simulink subsystem "Subsystem_TugAzimuth"  (R2023a)
settings: Solver=VariableStepAuto  StartTime=0.0  StopTime=10.0  RelTol=1e-3
model mask{PosAz=0}
  mask prompts: PosAz "Coordinates of azimuth: [x;y]"
settings Model: Creator=henni  LastModifiedBy=rkr021
settings DebuggingCC: UnconnectedInputMsg=warning  UnconnectedOutputMsg=warning  UnconnectedLineMsg=warning
settings ModelReferenceCC: EnableRefExpFcnMdlSchedulingChecks=on
settings RTWCC: DLArmComputeVersion=19.05

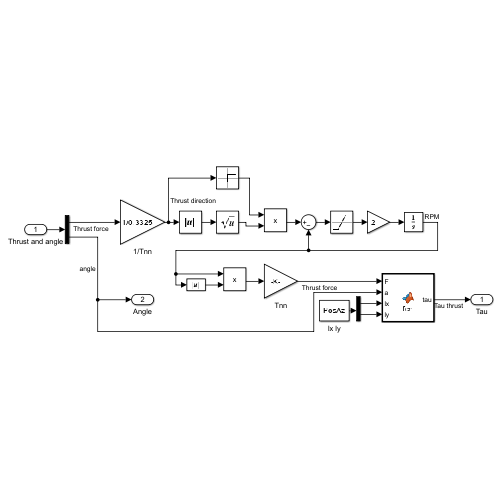
[thumbnail: Simulink's stored preview of the top-level diagram]
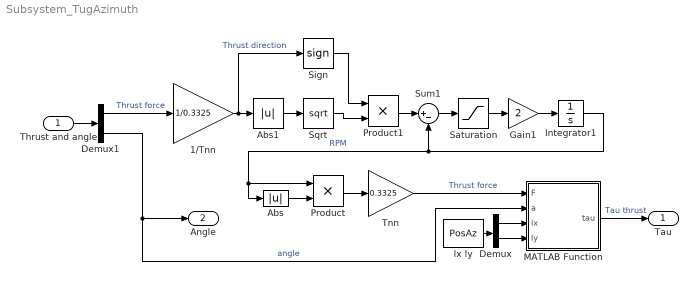
== system Subsystem_TugAzimuth ==
  Thrust and angle : Inport
  1/Tnn : Gain  Gain=1/0.3325
  Abs : Abs  SaturateOnIntegerOverflow=off
  Abs1 : Abs  SaturateOnIntegerOverflow=off
  Demux : Demux  Outputs=2
  Demux1 : Demux  Outputs=2
  Gain1 : Gain  Gain=2
  Integrator1 : Integrator  UpperSaturationLimit=100  LowerSaturationLimit=-100
  MATLAB Function : MATLAB Function  TreatAsAtomicUnit=on
  Product : Product
  Product1 : Product
  Saturation : Saturate  UpperLimit=50  LowerLimit=-50
  Sign : Signum
  Sqrt : Sqrt
  Sum1 : Sum  Inputs=|+-
  Tnn : Gain  Gain=0.3325
  lx ly : Constant  Value=PosAz
  Tau : Outport
  Angle : Outport  Port=2
  wires:
  Abs/1 -> Product/2
  Gain1/1 -> Integrator1/1
  Integrator1/1 -> Abs/1, Product/1, Sum1/2  "RPM"
  Saturation/1 -> Gain1/1
  Product/1 -> Tnn/1
  Sum1/1 -> Saturation/1
  MATLAB Function/1(tau) -> Tau/1  "Tau thrust"
  1/Tnn/1 -> Abs1/1, Sign/1  "Thrust direction"
  Sqrt/1 -> Product1/2
  Sign/1 -> Product1/1
  Product1/1 -> Sum1/1
  lx ly/1 -> Demux/1
  Demux/1 -> MATLAB Function/3(lx)
  Demux/2 -> MATLAB Function/4(ly)
  Demux1/1 -> 1/Tnn/1  "Thrust force"
  Demux1/2 -> Angle/1, MATLAB Function/2(a)  "angle"
  Thrust and angle/1 -> Demux1/1
  Abs1/1 -> Sqrt/1
  Tnn/1 -> MATLAB Function/1(F)  "Thrust force"

== matlab function Subsystem_TugAzimuth/MATLAB Function ==
  data: F input; tau output; a input; lx input; ly input
function tau = fcn(F, a, lx, ly)

tau = [cos(a); sin(a); -ly*cos(a)+lx*sin(a)]*F;
